simulink model "computed_torque"  (Simulink 8.8)
settings: Solver=FixedStepDiscrete  StartTime=0.0  StopTime=inf  FixedStep=0.01  RelTol=1e-3
InitFcn:
  | WBT_modelName = 'computed-torque';
  | WBT_wbiList = 'ROBOT_TORQUE_CONTROL_JOINTS_WITHOUT_PRONOSUP';
  | 
  | setenv('YARP_ROBOT_NAME','icubGazeboSim');
  | 
  | Dofs = 23;
  | ROBOT_DOF = Dofs;
  | Kp = 16*ones(Dofs, 1);
  | Kd = 8*ones(Dofs, 1);
libraries: WBToolboxLibrary x8
settings Model: SuppressorTable=22 serialization::archive 11 0 3 0 0 0 11 0  Creator=makaveli  LastModifiedBy=icub
settings DataIOCC: LimitDataPoints=off  SaveFormat=Dataset  SignalLoggingSaveFormat=Dataset
settings OptimizationCC: LifeSpan=auto
settings DebuggingCC: UnderspecifiedInitializationDetection=Simplified  MergeDetectMultiDrivingBlocksExec=error  FcnCallInpInsideContextMsg=error  StateNameClashWarn=none  SFUnexpectedBacktrackingDiag=error  SFNoUnconditionalDefaultTransitionDiag=error  SFExecutionAtInitializationDiag=warning
settings HardwareCC: ProdBitPerPointer=64  ProdBitPerSizeT=64  ProdBitPerPtrDiffT=64  ProdLargestAtomicFloat=Float  ProdIntDivRoundTo=Zero  ProdEndianess=LittleEndian  ProdWordSize=64  ProdHWDeviceType=Intel->x86-64 (Windows64)
settings ModelReferenceCC: PropagateSignalLabelsOutOfModel=on
settings GRTTargetCC: TargetLangStandard=C99 (ISO)  GeneratePreprocessorConditionals=Use local settings  CombineOutputUpdateFcns=on  GRTInterface=off
settings ConfigComp: CovMetricSettings=dwe  CovHtmlReporting=off  CovSaveCumulativeToWorkspaceVar=off  CovSaveSingleToWorkspaceVar=off  CovExternalEMLEnable=on

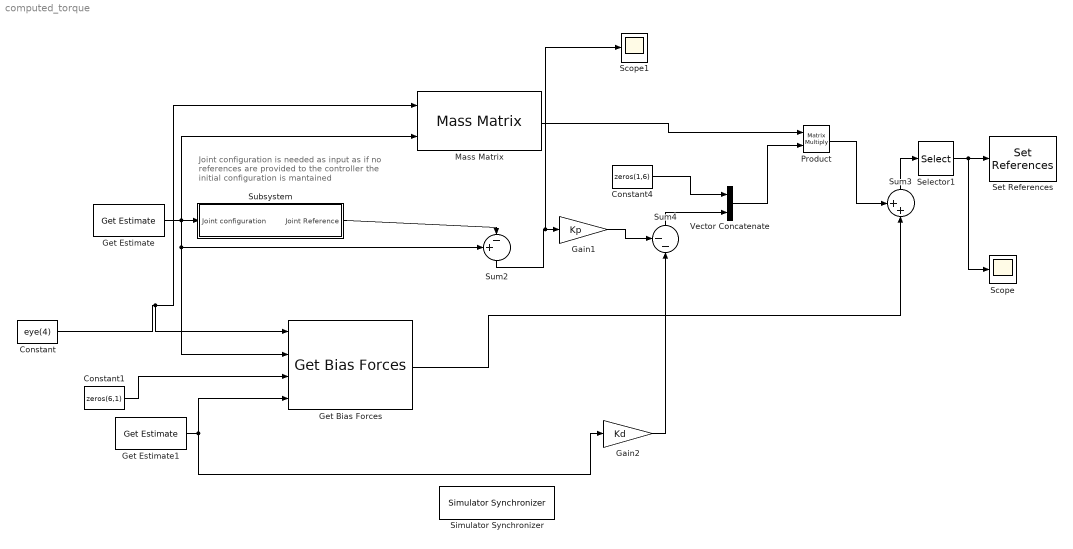
== system computed_torque ==
  note: Joint configuration is needed as input as
      | if no references are provided to the controller
      | the initial configuration is mantained
  Constant : Constant  Value=eye(4)
  Constant1 : Constant  Value=zeros(6,1)
  Constant4 : Constant  Value=zeros(1,6)
  Gain1 : Gain  Gain=Kp
  Gain2 : Gain  Gain=Kd
  Get Bias Forces : WBToolboxLibrary/wholeBodyModel/Dynamics/Get Bias Forces  robotName=WBT_robotName  localName=WBT_modelName  wbiFile=WBT_wbiFilename  wbiList=WBT_wbiList  explicitGravity=off
  Get Estimate : WBToolboxLibrary/wholeBodyStates/Get Estimate  estimateType=Joints Position  robotName=WBT_robotName  localName=WBT_modelName  wbiFile=WBT_wbiFilename  wbiList=WBT_wbiList
  Get Estimate1 : WBToolboxLibrary/wholeBodyStates/Get Estimate  estimateType=Joints Velocity  robotName=WBT_robotName  localName=WBT_modelName  wbiFile=WBT_wbiFilename  wbiList=WBT_wbiList
  Mass Matrix : WBToolboxLibrary/wholeBodyModel/Dynamics/Mass Matrix  robotName=WBT_robotName  localName=WBT_modelName  wbiFile=WBT_wbiFilename  wbiList=WBT_wbiList
  Product : Product  Multiplication=Matrix(*)
  Scope : Scope
  Scope1 : Scope
  Selector1 : Selector  InputPortWidth=ROBOT_DOF+6  IndexOptions=Index vector (dialog)  Indices=[7:ROBOT_DOF+6]  OutputSizes=1
  Set References : WBToolboxLibrary/wholeBodyActuators/Set References  controlType=Torque  fullOrSubControl=Full  controlledJoints=''  robotName=WBT_robotName  localName=WBT_modelName  wbiFile=WBT_wbiFilename  wbiList=WBT_wbiList
  Simulator Synchronizer : WBToolboxLibrary/Utilities/Simulator Synchronizer  period=0.01  serverPortName='/clock/rpc'  clientPortName='/WBT_synchronizer/rpc:o'
  Subsystem : Subsystem
  Sum2 : Sum  Inputs=+-|
  Sum3 : Sum  Inputs=++|
  Sum4 : Sum  Inputs=--|
  Vector Concatenate : Concatenate
  wires:
  Get Estimate/1 -> Mass Matrix/2, Get Bias Forces/2, Sum2/1, Subsystem/1(Joint configuration)
  Get Estimate1/1 -> Gain2/1, Get Bias Forces/4
  Subsystem/1(Joint Reference) -> Sum2/2
  Constant/1 -> Mass Matrix/1, Get Bias Forces/1
  Constant1/1 -> Get Bias Forces/3
  Product/1 -> Sum3/1
  Mass Matrix/1 -> Product/1
  Get Bias Forces/1 -> Sum3/2
  Vector Concatenate/1 -> Product/2
  Constant4/1 -> Vector Concatenate/1
  Sum2/1 -> Scope1/1, Gain1/1
  Sum4/1 -> Vector Concatenate/2
  Gain1/1 -> Sum4/1
  Gain2/1 -> Sum4/2
  Selector1/1 -> Scope/1, Set References/1
  Sum3/1 -> Selector1/1

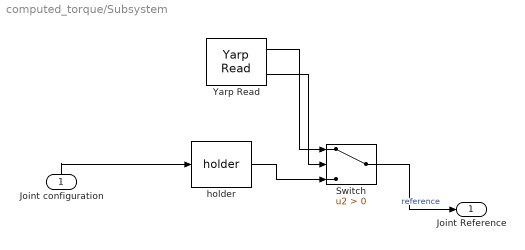
== system computed_torque/Subsystem ==
  Joint configuration : Inport
  Switch : Switch  Criteria=u2 > Threshold
  Yarp Read : WBToolboxLibrary/Utilities/Yarp Read  portName='/computed-torque/qDes:i'  signalSize=Dofs  blocking=off  timestamp=off  autoconnect=off  errorOnConnection=on
  "holder " : WBToolboxLibrary/Utilities/holder 
  Joint Reference : Outport
  wires:
  Switch/1 -> Joint Reference/1  "reference"
  "holder "/1 -> Switch/3
  Yarp Read/2 -> Switch/2
  Yarp Read/1 -> Switch/1
  Joint configuration/1 -> "holder "/1
